simulink model "a1_IEEE9_D"  (R2019a)
settings: Solver=ode23tb  StartTime=-1  StopTime=60  MaxStep=1/60  RelTol=1e-4  AbsTol=1e-3  EnableMultiTasking=on
InitFcn:
  | PSSMODEL=1;
  | MB=[1   0.2 30   1.25 40    12 160];
  | 
  | k=[8.3222    2.6014   19.0811    1.9818    3.6841   19.1783  240.6785    2.5684    4.3666   58.7391 7.6960   47.7975    8.7139  296.2463    2.7543    6.5051   47.7755    0.4780   35.4950   18.1866 94.2186]
  | k1=k(1);
  | k2=k(2);
  | k3=k(3);
  | k4=k(4);
  | k5=k(5);
  | k6=k(6);
  | k7=k(7);
  | k8=k(8);
  | k9=k(9);
  | k10=k(10);
  | k11=k(11);
  | k12=k(12);
  | k13=k(13);
  | k14=k(14);
  | k15=k(15);
  | k16=k(16);
  | k17=k(17);
  | k18=k(18);
  | k19=k(19);
  | k20=k(20);
  | k21=k(21);
values from neighbouring files (symbols this model uses):
  H1 = 2.444444*syn_s    (= 0.479111024)    [a1_IEEE9bus.m]    (also in calc_criticaltime9buses.m = 0.4888888; calc_criticaltime_10inertias.m = 2.444444; calc_nadir_support.m = 2.444444*syn_s; calc_nadirltime_10inertias.m = 2.444444)
  H2 = 5*syn_s    (= 0.98)    [a1_IEEE9bus.m]    (also in calc_criticaltime9buses.m = 1; calc_criticaltime_10inertias.m = 5; calc_nadir_support.m = 5*syn_s; calc_nadirltime_10inertias.m = 5)
  H3 = 5*syn_s    (= 0.98)    [a1_IEEE9bus.m]    (also in calc_criticaltime9buses.m = 1; calc_criticaltime_10inertias.m = 5; calc_nadir_support.m = 5*syn_s; calc_nadirltime_10inertias.m = 5)
  R1 = 0.05    [a1_IEEE9bus.m]    (also in calc_criticaltime9buses.m; calc_criticaltime_10inertias.m; calc_nadir_support.m; calc_nadirltime_10inertias.m)
  R2 = R1    (= 0.05)    [a1_IEEE9bus.m]    (also in calc_criticaltime9buses.m; calc_criticaltime_10inertias.m; calc_nadir_support.m; calc_nadirltime_10inertias.m)
  R3 = R2    (= 0.05)    [a1_IEEE9bus.m]    (also in calc_criticaltime9buses.m; calc_criticaltime_10inertias.m; calc_nadir_support.m; calc_nadirltime_10inertias.m)
  un = 0.30    (= 0.3)    [a1_IEEE9bus.m]    (also in calc_criticaltime9buses.m = 0.4; calc_criticaltime_10inertias.m; calc_nadir_support.m; calc_nadirltime_10inertias.m = 0.2)
undefined symbols (not defined in the file or in its folder): A, B, C, Dd, j
libraries: powerlib x53, sps_avr x3, powerlib_meascontrol x1, simulink x1
(part 1 of 2)
settings Model: Creator=jp536285  LastModifiedBy=Alejandro
settings SolverCC: AutoScaleAbsTol=off
settings DataIOCC: LimitDataPoints=on  SaveFormat=Array  ReturnWorkspaceOutputs=off
settings OptimizationCC: LifeSpan=inf
settings DebuggingCC: UnderspecifiedInitializationDetection=Classic  MergeDetectMultiDrivingBlocksExec=none  SolverPrmCheckMsg=warning  UnconnectedInputMsg=none  UnconnectedOutputMsg=none  UnconnectedLineMsg=none  StateNameClashWarn=warning  SFUnexpectedBacktrackingDiag=warning  SFNoUnconditionalDefaultTransitionDiag=warning  ArithmeticOperatorsInVariantConditions=warning
settings HardwareCC: ProdBitPerPointer=32  ProdBitPerSizeT=32  ProdBitPerPtrDiffT=32  ProdLargestAtomicFloat=None  ProdIntDivRoundTo=Undefined  ProdEndianess=Unspecified  ProdWordSize=32  ProdHWDeviceType=32-bit Generic
settings ModelReferenceCC: PropagateSignalLabelsOutOfModel=off
settings SFSimCC: SimUseLocalCustomCode=off
settings RTWCC: RTWUseLocalCustomCode=off
settings CodeAppCC: StateflowObjectComments=on
settings GRTTargetCC: TargetLangStandard=C89/C90 (ANSI)  GeneratePreprocessorConditionals=Disable all
settings ConfigComp: CovMetricSettings=dw  CovHtmlReporting=on  CovSaveCumulativeToWorkspaceVar=on  CovSaveSingleToWorkspaceVar=on  CovExternalEMLEnable=off
settings SimscapeCC: SimscapeNormalizeSystem=off

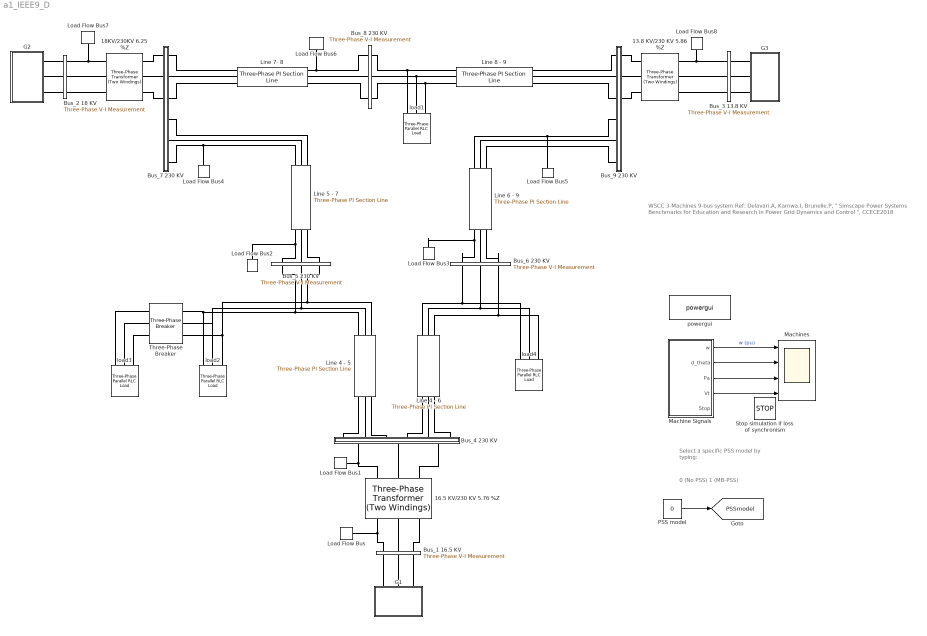
== system a1_IEEE9_D ==
  note: WSCC 3-Machines 9-bus system
      | Ref: Delavari.A, Kamwa.I, Brunelle.P, " Simscape Power Systems Benchmarks for Education
      | and Research in Power Grid Dynamics and Control ", CCECE2018
  note: Select a specific PSS model
      | by typing:
  note: 0  (No PSS)
      | 1  (MB-PSS)
  " Line 4 - 6" : powerlib/Elements/Three-Phase PI Section Line  LConnTagsString=a|b|c  RConnTagsString=A|B|C  Frequency=50  Resistances=[ 9.24e-2 9.24e-1]  Inductances=[ 1.33e-3 3.98e-3]  Capacitances=[8.14e-9 4.88e-9]  Length=97.336  mask(Three-Phase PI Section Line){}
      settings: SourceProductName=Simscape Electrical
      mask Display:
      | % This is a new mask on top of the base mask.
      | % Use "View base mask" link below to see the base mask.
      | patch([0.0 0.0 1 1 0.0 0.0 ],[0.4 0.7 0.7 0.4 0.4 0.7],[0 0 1]);
      | patch([0.4 0.4 0.42 0.42],[0.4 0.75 0.75 0.4],[1 0 0]);
      | patch([0.38 0.38 0.57 0.57],[0.7 0.75 0.75 0.7],[1 0 0]);
      | patch([0.53 0.53 0.55 0.55],[0.4 0.75 0.75 0.4],[1 0 0]);
  " Line 6 - 9" : powerlib/Elements/Three-Phase PI Section Line  LConnTagsString=a|b|c  RConnTagsString=A|B|C  Frequency=50  Resistances=[1.15 1.15e-1]  Inductances=[1.33e-3 3.98e-3]  Capacitances=[9.98e-9 5.99e-9]  Length=179.86  mask(Three-Phase PI Section Line){}
      settings: SourceProductName=Simscape Electrical
      mask Display:
      | % This is a new mask on top of the base mask.
      | % Use "View base mask" link below to see the base mask.
      | patch([0.0 0.0 1 1 0.0 0.0 ],[0.4 0.7 0.7 0.4 0.4 0.7],[0 0 1]);
      | patch([0.4 0.4 0.42 0.42],[0.4 0.75 0.75 0.4],[1 0 0]);
      | patch([0.38 0.38 0.57 0.57],[0.7 0.75 0.75 0.7],[1 0 0]);
      | patch([0.53 0.53 0.55 0.55],[0.4 0.75 0.75 0.4],[1 0 0]);
  13.8 KV/230 KV 5.86 %Z : powerlib/Elements/Three-Phase Transformer (Two Windings)  Winding1Connection=Yg  Winding2Connection=Yg  CoreType=Three single-phase transformers  SetSaturation=off  Hysteresis=off  DataFile='hysteresis'  SetInitialFlux=off  Measurements=None  UNITS=pu  NominalPower=[ 100e6 , 50 ]  Winding1=[ 13.8e3 , 1e-6 , 0 ]  Winding2=[ 230e3 , 1e-6, 0.0586 ]  Rm=500  Lm=500  L0=0.5  Saturation=[ 0,0 ; 0.0024,1.2 ; 1.0,1.52 ]  InitialFluxes=[ 0.8 , -0.8 , 0.7 ]  BreakLoop=off  DiscreteSolver=Trapezoidal iterative  DataType=off  TransfoNumber=1
      settings: SourceProductName=Simscape Electrical
  "16.5 KV/230 KV 5.76 %Z     " : powerlib/Elements/Three-Phase Transformer (Two Windings)  Winding1Connection=Yg  Winding2Connection=Yg  CoreType=Three single-phase transformers  SetSaturation=off  Hysteresis=off  DataFile='hysteresis'  SetInitialFlux=off  Measurements=None  UNITS=pu  NominalPower=[ 100e6 , 50 ]  Winding1=[ 16.5e3 , 1e-6, 0 ]  Winding2=[ 230e3 ,1e-6, 0.0576 ]  Rm=500  Lm=500  L0=0.5  Saturation=[ 0,0 ; 0.0024,1.2 ; 1.0,1.52 ]  InitialFluxes=[ 0.8 , -0.8 , 0.7 ]  BreakLoop=off  DiscreteSolver=Trapezoidal iterative  DataType=off  TransfoNumber=1
      settings: SourceProductName=Simscape Electrical
  18KV/230KV 6.25 %Z : powerlib/Elements/Three-Phase Transformer (Two Windings)  Winding1Connection=Yg  Winding2Connection=Yg  CoreType=Three single-phase transformers  SetSaturation=off  Hysteresis=off  DataFile='hysteresis'  SetInitialFlux=off  Measurements=None  UNITS=pu  NominalPower=[ 100e6 , 50 ]  Winding1=[ 18e3 , 1e-6 , 0]  Winding2=[ 230e3 , 1e-6, 0.0625 ]  Rm=500  Lm=500  L0=0.5  Saturation=[ 0,0 ; 0.0024,1.2 ; 1.0,1.52 ]  InitialFluxes=[ 0.8 , -0.8 , 0.7 ]  BreakLoop=off  DiscreteSolver=Trapezoidal iterative  DataType=off  TransfoNumber=1
      settings: SourceProductName=Simscape Electrical
  Bus_1 16.5 KV : powerlib/Measurements/Three-Phase V-I Measurement  VoltageMeasurement=phase-to-ground  SetLabelV=on  LabelV=Vabc_1  Vpu=on  VpuLL=off  CurrentMeasurement=yes  SetLabelI=on  LabelI=Iabc_1  Ipu=on  Pbase=100e6  Vbase=16.5e3  OutputType=Complex  PhasorSimulation=on  PSBequivalent=0
      settings: SourceProductName=Simscape Electrical
  Bus_2 18 KV : powerlib/Measurements/Three-Phase V-I Measurement  VoltageMeasurement=phase-to-ground  SetLabelV=on  LabelV=Vabc_2  Vpu=on  VpuLL=off  CurrentMeasurement=yes  SetLabelI=on  LabelI=Iabc_2  Ipu=on  Pbase=100e6  Vbase=18e3  OutputType=Complex  PhasorSimulation=on  PSBequivalent=0
      settings: SourceProductName=Simscape Electrical
  Bus_3 13.8 KV : powerlib/Measurements/Three-Phase V-I Measurement  VoltageMeasurement=phase-to-ground  SetLabelV=on  LabelV=Vabc_3  Vpu=on  VpuLL=off  CurrentMeasurement=yes  SetLabelI=on  LabelI=Iabc_3  Ipu=on  Pbase=100e6  Vbase=13.8e3  OutputType=Complex  PhasorSimulation=on  PSBequivalent=0
      settings: SourceProductName=Simscape Electrical
  Bus_4 230 KV : Subsystem
  Bus_5 230 KV : powerlib/Measurements/Three-Phase V-I Measurement  VoltageMeasurement=phase-to-ground  SetLabelV=on  LabelV=Vabc_5  Vpu=on  VpuLL=off  CurrentMeasurement=yes  SetLabelI=on  LabelI=Iabc_5  Ipu=on  Pbase=100e6  Vbase=230e3  OutputType=Complex  PhasorSimulation=on  PSBequivalent=0
      settings: SourceProductName=Simscape Electrical
  Bus_6 230 KV : powerlib/Measurements/Three-Phase V-I Measurement  VoltageMeasurement=phase-to-phase  SetLabelV=on  LabelV=Vabc_6  Vpu=off  VpuLL=on  CurrentMeasurement=yes  SetLabelI=on  LabelI=Iabc_6  Ipu=on  Pbase=100e6  Vbase=230e3  OutputType=Complex  PhasorSimulation=on  PSBequivalent=0
      settings: SourceProductName=Simscape Electrical
  Bus_7 230 KV : Subsystem
  Bus_8 230 KV : powerlib/Measurements/Three-Phase V-I Measurement  VoltageMeasurement=phase-to-phase  SetLabelV=on  LabelV=Vabc_8  Vpu=off  VpuLL=on  CurrentMeasurement=yes  SetLabelI=on  LabelI=Iabc_8  Ipu=on  Pbase=100e6  Vbase=230e3  OutputType=Complex  PhasorSimulation=on  PSBequivalent=0
      settings: SourceProductName=Simscape Electrical
  Bus_9 230 KV : Subsystem
  G1 : Subsystem
  G2 : Subsystem
  G3 : Subsystem
  "Line 4 - 5 " : powerlib/Elements/Three-Phase PI Section Line  LConnTagsString=a|b|c  RConnTagsString=A|B|C  Frequency=50  Resistances=[ 5.88e-2 5.88e-1]  Inductances=[ 1.33e-3 3.98e-3]  Capacitances=[9.81e-9 3.98e-3]  Length=89.93  mask(Three-Phase PI Section Line){}
      settings: SourceProductName=Simscape Electrical
      mask Display:
      | % This is a new mask on top of the base mask.
      | % Use "View base mask" link below to see the base mask.
      | patch([0.0 0.0 1 1 0.0 0.0 ],[0.4 0.7 0.7 0.4 0.4 0.7],[0 0 1]);
      | patch([0.4 0.4 0.42 0.42],[0.4 0.75 0.75 0.4],[1 0 0]);
      | patch([0.38 0.38 0.57 0.57],[0.7 0.75 0.75 0.7],[1 0 0]);
      | patch([0.53 0.53 0.55 0.55],[0.4 0.75 0.75 0.4],[1 0 0]);
  "Line 5 - 7 " : powerlib/Elements/Three-Phase PI Section Line  LConnTagsString=a|b|c  RConnTagsString=A|B|C  Frequency=50  Resistances=[9.94e-2 9.94e-1]  Inductances=[1.33e-3 3.98e-3]  Capacitances=[9.01e-9 5.41e-9]  Length=170.338  mask(Three-Phase PI Section Line){}
      settings: SourceProductName=Simscape Electrical
      mask Display:
      | % This is a new mask on top of the base mask.
      | % Use "View base mask" link below to see the base mask.
      | patch([0.0 0.0 1 1 0.0 0.0 ],[0.4 0.7 0.7 0.4 0.4 0.7],[0 0 1]);
      | patch([0.4 0.4 0.42 0.42],[0.4 0.75 0.75 0.4],[1 0 0]);
      | patch([0.38 0.38 0.57 0.57],[0.7 0.75 0.75 0.7],[1 0 0]);
      | patch([0.53 0.53 0.55 0.55],[0.4 0.75 0.75 0.4],[1 0 0]);
  Line 7- 8 : powerlib/Elements/Three-Phase PI Section Line  LConnTagsString=a|b|c  RConnTagsString=A|B|C  Frequency=50  Resistances=[5.9e-2 5.9e-1]  Inductances=[1.33e-3 3.98e-3]  Capacitances=[9.81e-9 5.89e-9]  Length=76.176  mask(Three-Phase PI Section Line){}
      settings: SourceProductName=Simscape Electrical
      mask Display:
      | % This is a new mask on top of the base mask.
      | % Use "View base mask" link below to see the base mask.
      | patch([0.0 0.0 1 1 0.0 0.0 ],[0.4 0.7 0.7 0.4 0.4 0.7],[0 0 1]);
      | patch([0.4 0.4 0.42 0.42],[0.4 0.75 0.75 0.4],[1 0 0]);
      | patch([0.38 0.38 0.57 0.57],[0.7 0.75 0.75 0.7],[1 0 0]);
      | patch([0.53 0.53 0.55 0.55],[0.4 0.75 0.75 0.4],[1 0 0]);
  Line 8 - 9 : powerlib/Elements/Three-Phase PI Section Line  LConnTagsString=a|b|c  RConnTagsString=A|B|C  Frequency=50  Resistances=[5.9e-2 5.9e-1]  Inductances=[1.33e-3 3.98e-3]  Capacitances=[9.83e-9 5.9e-9]  Length=106.649  mask(Three-Phase PI Section Line){}
      settings: SourceProductName=Simscape Electrical
      mask Display:
      | % This is a new mask on top of the base mask.
      | % Use "View base mask" link below to see the base mask.
      | patch([0.0 0.0 1 1 0.0 0.0 ],[0.4 0.7 0.7 0.4 0.4 0.7],[0 0 1]);
      | patch([0.4 0.4 0.42 0.42],[0.4 0.75 0.75 0.4],[1 0 0]);
      | patch([0.38 0.38 0.57 0.57],[0.7 0.75 0.75 0.7],[1 0 0]);
      | patch([0.53 0.53 0.55 0.55],[0.4 0.75 0.75 0.4],[1 0 0]);
  Load Flow Bus : powerlib/Measurements/Load Flow Bus  LConnTagsString=a  Phases=single  Connectors=on one side  ID=BUS_1  Vbase=16.5e3  Vref=1.04  Vangle=0  VLF=1.04  VLFb=1  VLFc=1  angleLF=0  angleLFb=0  angleLFc=0
      settings: AttributesFormatString=%<ID>\n%<Vbase>V\n%<VLF>pu\n%<angleLF>deg.  SourceProductName=Simscape Electrical
  Load Flow Bus1 : powerlib/Measurements/Load Flow Bus  LConnTagsString=a  Phases=single  Connectors=on one side  ID=BUS_4  Vbase=230e3  Vref=1  Vangle=0  VLF=1.021  VLFb=1  VLFc=1  angleLF=-2.239  angleLFb=0  angleLFc=0
      settings: AttributesFormatString=%<ID>\n%<Vbase>V\n%<VLF>pu\n%<angleLF>deg.  SourceProductName=Simscape Electrical
  Load Flow Bus2 : powerlib/Measurements/Load Flow Bus  LConnTagsString=a  Phases=single  Connectors=on one side  ID=BUS_5  Vbase=230e3  Vref=1  Vangle=0  VLF=0.9938  VLFb=1  VLFc=1  angleLF=-3.685  angleLFb=0  angleLFc=0
      settings: AttributesFormatString=%<ID>\n%<Vbase>V\n%<VLF>pu\n%<angleLF>deg.  SourceProductName=Simscape Electrical
  Load Flow Bus3 : powerlib/Measurements/Load Flow Bus  LConnTagsString=a  Phases=single  Connectors=on one side  ID=BUS_6  Vbase=230e3  Vref=1  Vangle=0  VLF=1.007  VLFb=1  VLFc=1  angleLF=-3.444  angleLFb=0  angleLFc=0
      settings: AttributesFormatString=%<ID>\n%<Vbase>V\n%<VLF>pu\n%<angleLF>deg.  SourceProductName=Simscape Electrical
  Load Flow Bus4 : powerlib/Measurements/Load Flow Bus  LConnTagsString=a  Phases=single  Connectors=on one side  ID=BUS_7  Vbase=230e3  Vref=1  Vangle=0  VLF=1.024  VLFb=1  VLFc=1  angleLF=2.693  angleLFb=0  angleLFc=0
      settings: AttributesFormatString=%<ID>\n%<Vbase>V\n%<VLF>pu\n%<angleLF>deg.  SourceProductName=Simscape Electrical
  Load Flow Bus5 : powerlib/Measurements/Load Flow Bus  LConnTagsString=a  Phases=single  Connectors=on one side  ID=BUS_9  Vbase=230e3  Vref=1  Vangle=0  VLF=1.029  VLFb=1  VLFc=1  angleLF=1.226  angleLFb=0  angleLFc=0
      settings: AttributesFormatString=%<ID>\n%<Vbase>V\n%<VLF>pu\n%<angleLF>deg.  SourceProductName=Simscape Electrical
  Load Flow Bus6 : powerlib/Measurements/Load Flow Bus  LConnTagsString=a  Phases=single  Connectors=on one side  ID=BUS_8  Vbase=230e3  Vref=1  Vangle=0  VLF=1.014  VLFb=1  VLFc=1  angleLF=0.2062  angleLFb=0  angleLFc=0
      settings: AttributesFormatString=%<ID>\n%<Vbase>V\n%<VLF>pu\n%<angleLF>deg.  SourceProductName=Simscape Electrical
  Load Flow Bus7 : powerlib/Measurements/Load Flow Bus  LConnTagsString=a  Phases=single  Connectors=on one side  ID=BUS_2  Vbase=18e3  Vref=1.025  Vangle=0  VLF=1.025  VLFb=1  VLFc=1  angleLF=8.256  angleLFb=0  angleLFc=0
      settings: AttributesFormatString=%<ID>\n%<Vbase>V\n%<VLF>pu\n%<angleLF>deg.  SourceProductName=Simscape Electrical
  Load Flow Bus8 : powerlib/Measurements/Load Flow Bus  LConnTagsString=a  Phases=single  Connectors=on one side  ID=BUS_3  Vbase=13.8e3  Vref=1.025  Vangle=0  VLF=1.025  VLFb=1  VLFc=1  angleLF=3.927  angleLFb=0  angleLFc=0
      settings: AttributesFormatString=%<ID>\n%<Vbase>V\n%<VLF>pu\n%<angleLF>deg.  SourceProductName=Simscape Electrical
  Machine Signals : Subsystem
  Machines : Scope  NumInputPorts=4
  PSS model : Constant  Value=0
  Stop simulation if loss of synchronism : Stop
  Three-Phase Breaker : powerlib/Elements/Three-Phase Breaker  InitialState=open  SwitchA=on  SwitchB=on  SwitchC=on  SwitchTimes=0  External=off  BreakerResistance=0.00001  SnubberResistance=1e9  SnubberCapacitance=inf  Measurements=None
      settings: SourceProductName=Simscape Electrical
  load1 : powerlib/Elements/Three-Phase Parallel RLC Load  LConnTagsString=A|B|C  Configuration=Y (grounded)  NominalVoltage=(230000)*1.01415  Vabc=[1e3 1e3 1e3]  Vabcp=[1e3 1e3 1e3]  NominalFrequency=50  UnbalancedPower=off  ActivePower=100e6  InductivePower=35e6  CapacitivePower=0  Pabc=[10e3 9e3 11e3]  QLabc=[100 90 110]  QCabc=[100 90 110]  Pabcp=[10e3 9e3 11e3]  QLabcp=[100 90 110]  QCabcp=[100 90 110]  Measurements=None  LoadType=constant PQ
      settings: SourceProductName=Simscape Electrical
  load2 : powerlib/Elements/Three-Phase Parallel RLC Load  LConnTagsString=A|B|C  Configuration=Y (grounded)  NominalVoltage=(230000)*0.993797  Vabc=[1e3 1e3 1e3]  Vabcp=[1e3 1e3 1e3]  NominalFrequency=50  UnbalancedPower=off  ActivePower=125e6  InductivePower=50e6  CapacitivePower=0  Pabc=[10e3 9e3 11e3]  QLabc=[100 90 110]  QCabc=[100 90 110]  Pabcp=[10e3 9e3 11e3]  QLabcp=[100 90 110]  QCabcp=[100 90 110]  Measurements=None  LoadType=constant PQ
      settings: SourceProductName=Simscape Electrical
  load3 : powerlib/Elements/Three-Phase Parallel RLC Load  LConnTagsString=A|B|C  Configuration=Y (grounded)  NominalVoltage=(230000)*0.993797  Vabc=[1e3 1e3 1e3]  Vabcp=[1e3 1e3 1e3]  NominalFrequency=50  UnbalancedPower=off  ActivePower=(315e6)*un  InductivePower=0  CapacitivePower=0  Pabc=[10e3 9e3 11e3]  QLabc=[100 90 110]  QCabc=[100 90 110]  Pabcp=[10e3 9e3 11e3]  QLabcp=[100 90 110]  QCabcp=[100 90 110]  Measurements=None  LoadType=constant PQ
      settings: SourceProductName=Simscape Electrical
  load4 : powerlib/Elements/Three-Phase Parallel RLC Load  LConnTagsString=A|B|C  Configuration=Y (grounded)  NominalVoltage=(230000)*1.00721  Vabc=[1e3 1e3 1e3]  Vabcp=[1e3 1e3 1e3]  NominalFrequency=50  UnbalancedPower=off  ActivePower=9e+07  InductivePower=3e+07  CapacitivePower=0  Pabc=[10e3 9e3 11e3]  QLabc=[100 90 110]  QCabc=[100 90 110]  Pabcp=[10e3 9e3 11e3]  QLabcp=[100 90 110]  QCabcp=[100 90 110]  Measurements=None  LoadType=constant PQ
      settings: SourceProductName=Simscape Electrical
  powergui : powerlib/powergui  Priority=1  SimulationMode=Phasor  SampleTime=50e-6  frequency=50  Iterations=50  frequencyindice=50  Pbase=10e7  ErrMax=1e-05  UnitsV=kV  UnitsW=MW  buscounter=0  FunctionMessages=off  echomessages=off  EnableUseOfTLC=off  CurrentSourceSwitches=off  DisableSnubberDevices=off  DisableRonSwitches=off  DisableVfSwitches=off  DisplayEquations=off  AutomaticDiscreteSolvers=off  SolverType=Tustin  Interpol=off  ExternalGateDelay=off  methode=off  Ts=0  x0status=steady  SPID=off  SwTol=0  HookPort=off  NonlinearTolerance=0  nMaxIteration=15  ContinueOnMaxIteration=off  RestoreLinks=warning  ResistiveCurrentMeasurement=off  Frange=[0:2:500]  Ylog=off  Xlog=on  ShowGrid=off  save=off  variable=ZData  structure=0  ZoomFFT=off  StartTime=0.0  cycles=1  DisplayStyle=1  fundamental=60  FreqAxis=off  MaxFrequency=1000  frequencyindicesteady=1  RmsSteady=1  display=off
      settings: SourceProductName=Simscape Electrical
  tag scope: PSSmodel=global
  wires:
  Machine Signals/1(w) -> Machines/1  "w (pu)"
  Machine Signals/2(d_theta) -> Machines/2
  Machine Signals/3(Pa) -> Machines/3
  Machine Signals/4(Vt) -> Machines/4
  PSS model/1 -> [PSSmodel]
  connections:
  G2/LConn2 -- Bus_2 18 KV/LConn2
  18KV/230KV 6.25 %Z/LConn2 -- Bus_2 18 KV/RConn2
  18KV/230KV 6.25 %Z/RConn2 -- Bus_7 230 KV/LConn2
  Bus_2 18 KV/RConn1 -- 18KV/230KV 6.25 %Z/LConn1 -- Load Flow Bus7/LConn1
  Bus_2 18 KV/RConn3 -- 18KV/230KV 6.25 %Z/LConn3
  Bus_7 230 KV/LConn1 -- 18KV/230KV 6.25 %Z/RConn1
  18KV/230KV 6.25 %Z/RConn3 -- Bus_7 230 KV/LConn3
  Load Flow Bus8/LConn1 -- 13.8 KV/230 KV 5.86 %Z/LConn1 -- Bus_3 13.8 KV/LConn1
  13.8 KV/230 KV 5.86 %Z/LConn2 -- Bus_3 13.8 KV/LConn2
  13.8 KV/230 KV 5.86 %Z/LConn3 -- Bus_3 13.8 KV/LConn3
  Bus_1 16.5 KV/LConn1 -- Load Flow Bus/LConn1 -- "16.5 KV/230 KV 5.76 %Z     "/LConn1
  Bus_1 16.5 KV/LConn3 -- "16.5 KV/230 KV 5.76 %Z     "/LConn3
  Bus_1 16.5 KV/LConn2 -- "16.5 KV/230 KV 5.76 %Z     "/LConn2
  13.8 KV/230 KV 5.86 %Z/RConn1 -- Bus_9 230 KV/RConn1
  13.8 KV/230 KV 5.86 %Z/RConn2 -- Bus_9 230 KV/RConn2
  13.8 KV/230 KV 5.86 %Z/RConn3 -- Bus_9 230 KV/RConn3
  Bus_4 230 KV/LConn1 -- "16.5 KV/230 KV 5.76 %Z     "/RConn1 -- Load Flow Bus1/LConn1
  Bus_4 230 KV/LConn2 -- "16.5 KV/230 KV 5.76 %Z     "/RConn2
  Line 8 - 9/LConn1 -- load1/LConn1 -- Bus_8 230 KV/LConn1
  Bus_8 230 KV/LConn2 -- load1/LConn2 -- Line 8 - 9/LConn2
  Line 8 - 9/LConn3 -- load1/LConn3 -- Bus_8 230 KV/LConn3
  "16.5 KV/230 KV 5.76 %Z     "/RConn3 -- Bus_4 230 KV/LConn3
  "Line 4 - 5 "/LConn1 -- Bus_5 230 KV/RConn1 -- load2/LConn1 -- Three-Phase Breaker/RConn1
  "Line 4 - 5 "/LConn2 -- Three-Phase Breaker/RConn2 -- load2/LConn2 -- Bus_5 230 KV/RConn2
  "Line 4 - 5 "/LConn3 -- Bus_5 230 KV/RConn3 -- Three-Phase Breaker/RConn3 -- load2/LConn3
  " Line 4 - 6"/LConn1 -- load4/LConn1 -- Bus_6 230 KV/RConn1
  " Line 4 - 6"/LConn2 -- load4/LConn2 -- Bus_6 230 KV/RConn2
  " Line 4 - 6"/LConn3 -- load4/LConn3 -- Bus_6 230 KV/RConn3
  Line 7- 8/LConn1 -- Bus_7 230 KV/RConn1
  Line 7- 8/LConn2 -- Bus_7 230 KV/RConn2
  Bus_7 230 KV/RConn3 -- Line 7- 8/LConn3
  Bus_8 230 KV/RConn1 -- Load Flow Bus6/LConn1 -- Line 7- 8/RConn1
  Line 7- 8/RConn2 -- Bus_8 230 KV/RConn2
  Line 7- 8/RConn3 -- Bus_8 230 KV/RConn3
  Line 8 - 9/RConn2 -- Bus_9 230 KV/LConn2
  Line 8 - 9/RConn1 -- Bus_9 230 KV/LConn1
  Line 8 - 9/RConn3 -- Bus_9 230 KV/LConn3
  "Line 5 - 7 "/RConn1 -- Bus_5 230 KV/LConn1 -- Load Flow Bus2/LConn1
  "Line 5 - 7 "/RConn2 -- Bus_5 230 KV/LConn2
  "Line 5 - 7 "/RConn3 -- Bus_5 230 KV/LConn3
  "Line 5 - 7 "/LConn1 -- Load Flow Bus4/LConn1 -- Bus_7 230 KV/RConn6
  "Line 5 - 7 "/LConn2 -- Bus_7 230 KV/RConn5
  "Line 5 - 7 "/LConn3 -- Bus_7 230 KV/RConn4
  " Line 6 - 9"/RConn1 -- Load Flow Bus5/LConn1 -- Bus_9 230 KV/LConn4
  Bus_9 230 KV/LConn5 -- " Line 6 - 9"/RConn2
  Bus_6 230 KV/LConn1 -- Load Flow Bus3/LConn1 -- " Line 6 - 9"/LConn1
  Bus_6 230 KV/LConn2 -- " Line 6 - 9"/LConn2
  Bus_6 230 KV/LConn3 -- " Line 6 - 9"/LConn3
  " Line 6 - 9"/RConn3 -- Bus_9 230 KV/LConn6
  "Line 4 - 5 "/RConn2 -- Bus_4 230 KV/RConn2
  "Line 4 - 5 "/RConn1 -- Bus_4 230 KV/RConn1
  "Line 4 - 5 "/RConn3 -- Bus_4 230 KV/RConn3
  " Line 4 - 6"/RConn2 -- Bus_4 230 KV/RConn5
  " Line 4 - 6"/RConn1 -- Bus_4 230 KV/RConn4
  " Line 4 - 6"/RConn3 -- Bus_4 230 KV/RConn6
  G3/LConn1 -- Bus_3 13.8 KV/RConn1
  G3/LConn2 -- Bus_3 13.8 KV/RConn2
  G3/LConn3 -- Bus_3 13.8 KV/RConn3
  G2/LConn3 -- Bus_2 18 KV/LConn3
  G2/LConn1 -- Bus_2 18 KV/LConn1
  G1/LConn1 -- Bus_1 16.5 KV/RConn1
  G1/LConn2 -- Bus_1 16.5 KV/RConn2
  G1/LConn3 -- Bus_1 16.5 KV/RConn3
  load3/LConn1 -- Three-Phase Breaker/LConn1
  load3/LConn2 -- Three-Phase Breaker/LConn2
  load3/LConn3 -- Three-Phase Breaker/LConn3

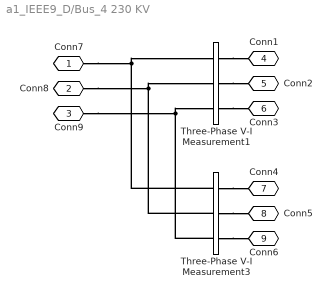
== system a1_IEEE9_D/Bus_4 230 KV ==
  Three-Phase V-I Measurement1 : powerlib/Measurements/Three-Phase V-I Measurement  VoltageMeasurement=phase-to-ground  SetLabelV=on  LabelV=Vabc_45  Vpu=on  VpuLL=off  CurrentMeasurement=yes  SetLabelI=on  LabelI=Iabc_45  Ipu=on  Pbase=100e6  Vbase=230e3  OutputType=Complex  PhasorSimulation=on  PSBequivalent=0
      settings: SourceProductName=Simscape Electrical
  Three-Phase V-I Measurement3 : powerlib/Measurements/Three-Phase V-I Measurement  VoltageMeasurement=phase-to-ground  SetLabelV=on  LabelV=Vabc_46  Vpu=on  VpuLL=off  CurrentMeasurement=yes  SetLabelI=on  LabelI=Iabc_46  Ipu=on  Pbase=100e6  Vbase=230e3  OutputType=Complex  PhasorSimulation=on  PSBequivalent=0
      settings: SourceProductName=Simscape Electrical
  Conn7 : PMIOPort  Side=Left
  Conn8 : PMIOPort  Port=2  Side=Left
  Conn9 : PMIOPort  Port=3  Side=Left
  Conn1 : PMIOPort  Port=4  Side=Right
  Conn2 : PMIOPort  Port=5  Side=Right
  Conn3 : PMIOPort  Port=6  Side=Right
  Conn4 : PMIOPort  Port=7  Side=Right
  Conn5 : PMIOPort  Port=8  Side=Right
  Conn6 : PMIOPort  Port=9  Side=Right
  connections:
  Three-Phase V-I Measurement3/LConn3 -- Conn9/RConn1 -- Three-Phase V-I Measurement1/LConn3
  Three-Phase V-I Measurement3/LConn2 -- Conn8/RConn1 -- Three-Phase V-I Measurement1/LConn2
  Three-Phase V-I Measurement3/LConn1 -- Conn7/RConn1 -- Three-Phase V-I Measurement1/LConn1
  Three-Phase V-I Measurement3/RConn3 -- Conn6/RConn1
  Three-Phase V-I Measurement1/RConn3 -- Conn3/RConn1
  Three-Phase V-I Measurement1/RConn1 -- Conn1/RConn1
  Three-Phase V-I Measurement1/RConn2 -- Conn2/RConn1
  Three-Phase V-I Measurement3/RConn1 -- Conn4/RConn1
  Three-Phase V-I Measurement3/RConn2 -- Conn5/RConn1

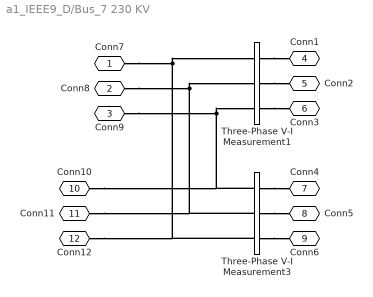
== system a1_IEEE9_D/Bus_7 230 KV ==
  Three-Phase V-I Measurement1 : powerlib/Measurements/Three-Phase V-I Measurement  VoltageMeasurement=phase-to-ground  SetLabelV=on  LabelV=Vabc_7  Vpu=on  VpuLL=off  CurrentMeasurement=yes  SetLabelI=on  LabelI=Iabc_7  Ipu=on  Pbase=100e6  Vbase=230e3  OutputType=Complex  PhasorSimulation=on  PSBequivalent=0
      settings: SourceProductName=Simscape Electrical
  Three-Phase V-I Measurement3 : powerlib/Measurements/Three-Phase V-I Measurement  VoltageMeasurement=phase-to-ground  SetLabelV=on  LabelV=Vab  Vpu=on  VpuLL=off  CurrentMeasurement=yes  SetLabelI=on  LabelI=Iab  Ipu=on  Pbase=100e6  Vbase=230e3  OutputType=Complex  PhasorSimulation=on  PSBequivalent=0
      settings: SourceProductName=Simscape Electrical
  Conn7 : PMIOPort  Side=Left
  Conn8 : PMIOPort  Port=2  Side=Left
  Conn9 : PMIOPort  Port=3  Side=Left
  Conn1 : PMIOPort  Port=4  Side=Right
  Conn2 : PMIOPort  Port=5  Side=Right
  Conn3 : PMIOPort  Port=6  Side=Right
  Conn4 : PMIOPort  Port=7  Side=Right
  Conn5 : PMIOPort  Port=8  Side=Right
  Conn6 : PMIOPort  Port=9  Side=Right
  Conn10 : PMIOPort  Port=10  Side=Left
  Conn11 : PMIOPort  Port=11  Side=Left
  Conn12 : PMIOPort  Port=12  Side=Left
  connections:
  Three-Phase V-I Measurement3/RConn2 -- Conn5/RConn1
  Three-Phase V-I Measurement3/RConn1 -- Conn4/RConn1
  Three-Phase V-I Measurement1/RConn2 -- Conn2/RConn1
  Three-Phase V-I Measurement1/RConn1 -- Conn1/RConn1
  Three-Phase V-I Measurement1/RConn3 -- Conn3/RConn1
  Three-Phase V-I Measurement3/RConn3 -- Conn6/RConn1
  Conn7/RConn1 -- Three-Phase V-I Measurement3/LConn3 -- Conn12/RConn1 -- Three-Phase V-I Measurement1/LConn1
  Conn8/RConn1 -- Three-Phase V-I Measurement3/LConn2 -- Conn11/RConn1 -- Three-Phase V-I Measurement1/LConn2
  Conn9/RConn1 -- Conn10/RConn1 -- Three-Phase V-I Measurement3/LConn1 -- Three-Phase V-I Measurement1/LConn3

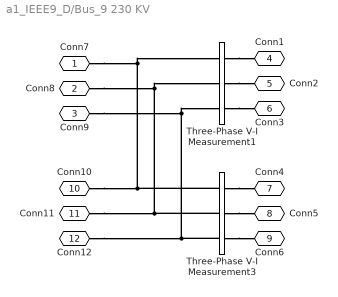
== system a1_IEEE9_D/Bus_9 230 KV ==
  Three-Phase V-I Measurement1 : powerlib/Measurements/Three-Phase V-I Measurement  VoltageMeasurement=phase-to-ground  SetLabelV=on  LabelV=Vabc_9  Vpu=on  VpuLL=off  CurrentMeasurement=yes  SetLabelI=on  LabelI=Iabc_9  Ipu=on  Pbase=100e6  Vbase=230e3  OutputType=Complex  PhasorSimulation=on  PSBequivalent=0
      settings: SourceProductName=Simscape Electrical
  Three-Phase V-I Measurement3 : powerlib/Measurements/Three-Phase V-I Measurement  VoltageMeasurement=phase-to-ground  SetLabelV=on  LabelV=Vabc  Vpu=on  VpuLL=off  CurrentMeasurement=yes  SetLabelI=on  LabelI=Iabc  Ipu=on  Pbase=100e6  Vbase=230e3  OutputType=Complex  PhasorSimulation=on  PSBequivalent=0
      settings: SourceProductName=Simscape Electrical
  Conn7 : PMIOPort  Side=Left
  Conn8 : PMIOPort  Port=2  Side=Left
  Conn9 : PMIOPort  Port=3  Side=Left
  Conn1 : PMIOPort  Port=4  Side=Right
  Conn2 : PMIOPort  Port=5  Side=Right
  Conn3 : PMIOPort  Port=6  Side=Right
  Conn4 : PMIOPort  Port=7  Side=Right
  Conn5 : PMIOPort  Port=8  Side=Right
  Conn6 : PMIOPort  Port=9  Side=Right
  Conn10 : PMIOPort  Port=10  Side=Left
  Conn11 : PMIOPort  Port=11  Side=Left
  Conn12 : PMIOPort  Port=12  Side=Left
  connections:
  Conn12/RConn1 -- Three-Phase V-I Measurement3/LConn3 -- Conn9/RConn1 -- Three-Phase V-I Measurement1/LConn3
  Conn11/RConn1 -- Three-Phase V-I Measurement3/LConn2 -- Conn8/RConn1 -- Three-Phase V-I Measurement1/LConn2
  Conn10/RConn1 -- Three-Phase V-I Measurement3/LConn1 -- Conn7/RConn1 -- Three-Phase V-I Measurement1/LConn1
  Three-Phase V-I Measurement3/RConn3 -- Conn6/RConn1
  Three-Phase V-I Measurement1/RConn3 -- Conn3/RConn1
  Three-Phase V-I Measurement1/RConn1 -- Conn1/RConn1
  Three-Phase V-I Measurement1/RConn2 -- Conn2/RConn1
  Three-Phase V-I Measurement3/RConn1 -- Conn4/RConn1
  Three-Phase V-I Measurement3/RConn2 -- Conn5/RConn1

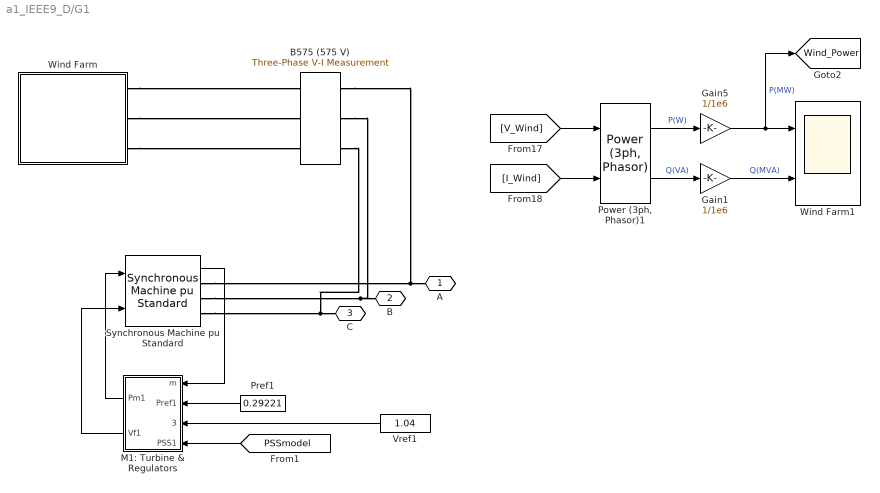
== system a1_IEEE9_D/G1 ==
  B575 (575 V) : powerlib/Measurements/Three-Phase V-I Measurement  VoltageMeasurement=phase-to-ground  SetLabelV=on  LabelV=V_Wind  Vpu=off  VpuLL=off  CurrentMeasurement=yes  SetLabelI=on  LabelI=I_Wind  Ipu=off  Pbase=6*1.5e6/0.9  Vbase=575  OutputType=Complex  PhasorSimulation=on  PSBequivalent=0
      settings: SourceProductName=Simscape Electrical
  Gain1 : Gain  Gain=1/1e6
  Gain5 : Gain  Gain=1/1e6
  M1: Turbine & Regulators : Subsystem
  "Power (3ph, Phasor)1" : powerlib_meascontrol/Measurements/Power (3ph, Phasor)
      settings: SourceProductName=Simscape Electrical  SourceProductBaseCode=PS
  Pref1 : Constant  Value=0.29221
  Synchronous Machine pu Standard : powerlib/Machines/Synchronous Machine pu Standard  PresetModel=No  MechanicalLoad=Mechanical power Pm  ShowDetailedParameters=on  RotorType=Round  Units=per unit standard parameters  MeasurementBus=off  NominalParameters="[247.5e6  16500   50 ]"  Reactances1=[ 1.81, 0.3, 0.23, 1.76, 0.65, 0.25, 0.15 ]  Reactances2=[1.146 .0608 .25 0.0969*10 0.0969 .25 .025]  dAxisTimeConstants=Open-circuit  qAxisTimeConstants=Open-circuit  TimeConstants1=[8.96 0.3 0.31 0.05]  TimeConstants2=[ 8.0, 0.03, 1.0, 0.07 ]  TimeConstants3="[  4.49  0.0681  0.0513  ]"  TimeConstants4=[ 8.0, 0.03, 0.3371, 0.0295 ]  TimeConstants5=[ 1.01, 0.053, 0.1 ]  TimeConstants6=[ 1.3201, 0.023, 1.0, 0.07 ]  TimeConstants7=[0.012 0.003 0.003]  TimeConstants8=[ 1.3201, 0.0231, 0.3371, 0.0295 ]  StatorResistance=0.0025  Mechanical="[ H1  0  4]"  PolePairs=20  InitialConditions=[0 -68.9621 0.312855 0.312855 0.312855 -26.1902 -146.19 93.8098 1.38688]  SetSaturation=off  Saturation=[0.6404,0.7127,0.8441,0.9214,0.9956,1.082,1.19,1.316,1.457;0.7,0.7698,0.8872,0.9466,0.9969,1.046,1.1,1.151,1.201]  LoadFlowParameters=[2 72000000 0 0 0]  TsPowergui=0  TsBlock=-1  IterativeModel=Trapezoidal non iterative  IterativeDiscreteModel=Trapezoidal non iterative  BusType=swing  Pref=0  Qref=0  Qmin=-inf  Qmax=inf  PLF=0  QLF=0
      settings: SourceProductName=Simscape Electrical
  Vref1 : Constant  Value=1.04
  Wind Farm : Subsystem
  Wind Farm1 : Scope  NumInputPorts=2
  A : PMIOPort  Side=Left
  B : PMIOPort  Port=2  Side=Left
  C : PMIOPort  Port=3  Side=Left
  tag scope: Wind_Power=global
  wires:
  Pref1/1 -> M1: Turbine & Regulators/2(Pref1)
  [PSSmodel] -> M1: Turbine & Regulators/4(PSS1)
  M1: Turbine & Regulators/1(Pm1) -> Synchronous Machine pu Standard/1
  M1: Turbine & Regulators/2(Vf1) -> Synchronous Machine pu Standard/2
  Vref1/1 -> M1: Turbine & Regulators/3(Vref1)
  Synchronous Machine pu Standard/1 -> M1: Turbine & Regulators/1(m)
  [V_Wind] -> "Power (3ph, Phasor)1"/1
  "Power (3ph, Phasor)1"/2 -> Gain1/1  "Q(VA)"
  Gain1/1 -> Wind Farm1/2  "Q(MVA)"
  "Power (3ph, Phasor)1"/1 -> Gain5/1  "P(W)"
  [I_Wind] -> "Power (3ph, Phasor)1"/2
  Gain5/1 -> [Wind_Power], Wind Farm1/1  "P(MW)"
  connections:
  Synchronous Machine pu Standard/RConn1 -- B575 (575 V)/RConn1 -- A/RConn1
  Synchronous Machine pu Standard/RConn2 -- B575 (575 V)/RConn2 -- B/RConn1
  Synchronous Machine pu Standard/RConn3 -- B575 (575 V)/RConn3 -- C/RConn1
  Wind Farm/RConn1 -- B575 (575 V)/LConn1
  Wind Farm/RConn2 -- B575 (575 V)/LConn2
  Wind Farm/RConn3 -- B575 (575 V)/LConn3

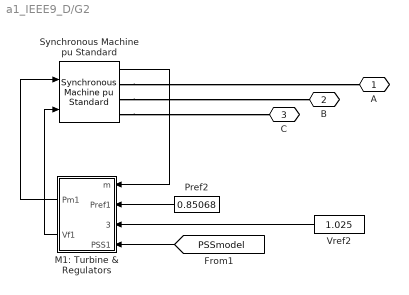
== system a1_IEEE9_D/G2 ==
  M1: Turbine & Regulators : Subsystem
  Pref2 : Constant  Value=0.85068
  Synchronous Machine pu Standard : powerlib/Machines/Synchronous Machine pu Standard  PresetModel=No  MechanicalLoad=Mechanical power Pm  ShowDetailedParameters=on  RotorType=Round  Units=per unit standard parameters  MeasurementBus=off  NominalParameters="[192e6  18000   50 ]"  Reactances1=[0.8958 .1198 .25 1.7 .8645 .1969 .220]  Reactances2=[2.24 0.17 0.12 1.02 0.13 0.08]  dAxisTimeConstants=Open-circuit  qAxisTimeConstants=Open-circuit  TimeConstants1="[ 4.4849  0.0681  0.1  ]"  TimeConstants2=[6 .03 .535 .05]  TimeConstants3="[  4.49  0.0681  0.0513  ]"  TimeConstants4=[ 8.0, 0.03, 0.3371, 0.0295 ]  TimeConstants5=[ 1.01, 0.053, 0.1 ]  TimeConstants6=[ 1.3201, 0.023, 1.0, 0.07 ]  TimeConstants7=[0.012 0.003 0.003]  TimeConstants8=[ 1.3201, 0.0231, 0.3371, 0.0295 ]  StatorResistance=0.0025  Mechanical="[ H2  0  4]"  PolePairs=20  InitialConditions=[0 -30.0411 0.82975 0.82975 0.82975 4.813 -115.187 124.813 1.24637]  SetSaturation=off  Saturation=[0.6404,0.7127,0.8441,0.9214,0.9956,1.082,1.19,1.316,1.457;0.7,0.7698,0.8872,0.9466,0.9969,1.046,1.1,1.151,1.201]  LoadFlowParameters=[1,0,0,0,0]  TsPowergui=0  TsBlock=-1  IterativeModel=Trapezoidal non iterative  IterativeDiscreteModel=Trapezoidal non iterative  BusType=PV  Pref=163e6  Qref=0  Qmin=-inf  Qmax=inf  PLF=0  QLF=0
      settings: SourceProductName=Simscape Electrical
  Vref2 : Constant  Value=1.025
  A : PMIOPort  Side=Left
  B : PMIOPort  Port=2  Side=Left
  C : PMIOPort  Port=3  Side=Left
  wires:
  Pref2/1 -> M1: Turbine & Regulators/2(Pref1)
  [PSSmodel] -> M1: Turbine & Regulators/4(PSS1)
  M1: Turbine & Regulators/1(Pm1) -> Synchronous Machine pu Standard/1
  M1: Turbine & Regulators/2(Vf1) -> Synchronous Machine pu Standard/2
  Synchronous Machine pu Standard/1 -> M1: Turbine & Regulators/1(m)
  Vref2/1 -> M1: Turbine & Regulators/3(Vref1)
  connections:
  Synchronous Machine pu Standard/RConn1 -- A/RConn1
  Synchronous Machine pu Standard/RConn2 -- B/RConn1
  Synchronous Machine pu Standard/RConn3 -- C/RConn1

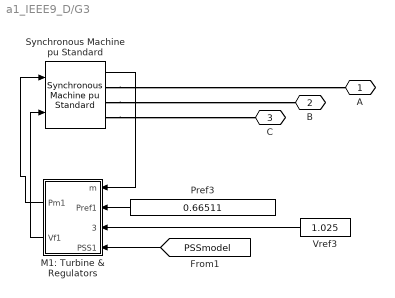
== system a1_IEEE9_D/G3 ==
  M1: Turbine & Regulators : Subsystem
  Pref3 : Constant  Value=0.66511
  Synchronous Machine pu Standard : powerlib/Machines/Synchronous Machine pu Standard  PresetModel=No  MechanicalLoad=Mechanical power Pm  ShowDetailedParameters=on  RotorType=Round  Units=per unit standard parameters  MeasurementBus=off  NominalParameters="[128e6  13800   50 ]"  Reactances1=[1.3125 .1813 .25 1.2578 .25 .25 .246]  Reactances2=[2.24 0.17 0.12 1.02 0.13 0.08]  dAxisTimeConstants=Open-circuit  qAxisTimeConstants=Open-circuit  TimeConstants1="[ 4.4849  0.0681  0.1  ]"  TimeConstants2=[5.89 .03 .6 .05]  TimeConstants3="[  4.49  0.0681  0.0513  ]"  TimeConstants4=[ 8.0, 0.03, 0.3371, 0.0295 ]  TimeConstants5=[ 1.01, 0.053, 0.1 ]  TimeConstants6=[ 1.3201, 0.023, 1.0, 0.07 ]  TimeConstants7=[0.012 0.003 0.003]  TimeConstants8=[ 1.3201, 0.0231, 0.3371, 0.0295 ]  StatorResistance=0.0025  Mechanical="[ H3  0  4]"  PolePairs=20  InitialConditions=[0 -46.4509 0.648737 0.648737 0.648737 6.89632 -113.104 126.896 1.29912]  SetSaturation=off  Saturation=[0.6404,0.7127,0.8441,0.9214,0.9956,1.082,1.19,1.316,1.457;0.7,0.7698,0.8872,0.9466,0.9969,1.046,1.1,1.151,1.201]  LoadFlowParameters=[1,0,0,0,0]  TsPowergui=0  TsBlock=-1  IterativeModel=Trapezoidal non iterative  IterativeDiscreteModel=Trapezoidal non iterative  BusType=PV  Pref=85e6  Qref=0  Qmin=-inf  Qmax=inf  PLF=0  QLF=0
      settings: SourceProductName=Simscape Electrical
  Vref3 : Constant  Value=1.025
  A : PMIOPort  Side=Left
  B : PMIOPort  Port=2  Side=Left
  C : PMIOPort  Port=3  Side=Left
  wires:
  Vref3/1 -> M1: Turbine & Regulators/3(Vref1)
  Synchronous Machine pu Standard/1 -> M1: Turbine & Regulators/1(m)
  M1: Turbine & Regulators/2(Vf1) -> Synchronous Machine pu Standard/2
  M1: Turbine & Regulators/1(Pm1) -> Synchronous Machine pu Standard/1
  [PSSmodel] -> M1: Turbine & Regulators/4(PSS1)
  Pref3/1 -> M1: Turbine & Regulators/2(Pref1)
  connections:
  Synchronous Machine pu Standard/RConn3 -- C/RConn1
  Synchronous Machine pu Standard/RConn2 -- B/RConn1
  Synchronous Machine pu Standard/RConn1 -- A/RConn1

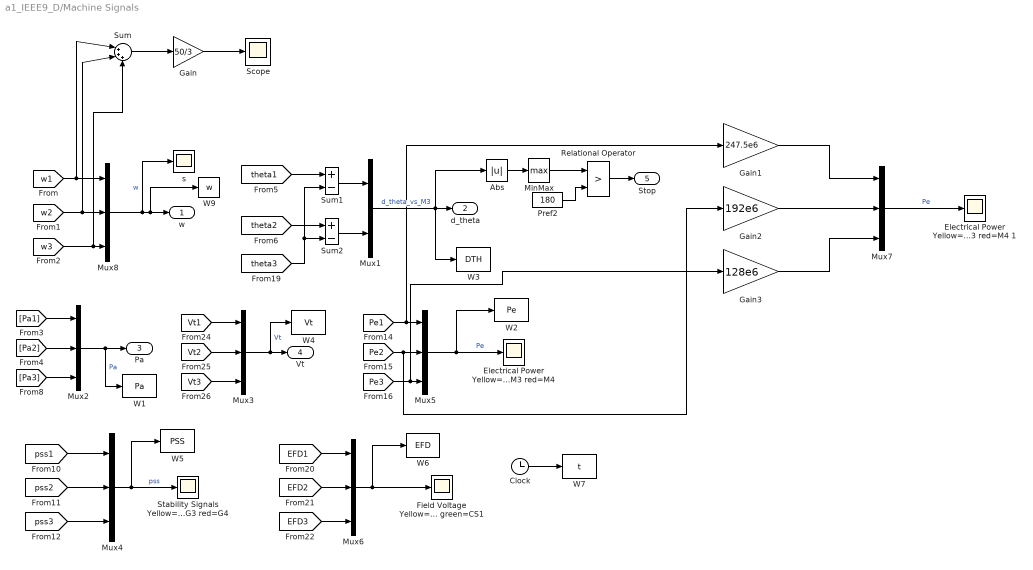
== system a1_IEEE9_D/Machine Signals ==
  Abs : Abs  SaturateOnIntegerOverflow=on
  Clock : Clock
  "Electrical Power Yellow=M1 mag=M2 cyan=M3 red=M4 " : Scope
  Electrical Power Yellow=M1 mag=M2 cyan=M3 red=M4 1 : Scope
  Field Voltage Yellow=G1 mag=G2 cyan=G3 red=G4 green=CS1 : Scope
  Gain : Gain  Gain=50/3
  Gain1 : Gain  Gain=247.5e6
  Gain2 : Gain  Gain=192e6
  Gain3 : Gain  Gain=128e6
  MinMax : MinMax  Function=max  SaturateOnIntegerOverflow=on  InputSameDT=on
  Mux1 : Mux  Inputs=2
  Mux{2..8} (7 alike) : Mux  Inputs=3
  Pref2 : Constant  Value=180
  Relational Operator : RelationalOperator  Operator=>  RndMeth=Nearest  InputSameDT=on
  Scope : Scope
  "Stability Signals Yellow=G1 mag=G2 cyan=G3 red=G4 " : Scope
  Sum : Sum  Inputs=|+++
  Sum1 : Sum  Inputs=+-  SaturateOnIntegerOverflow=on  InputSameDT=on  OutDataTypeStr=Inherit: Same as first input
  Sum2 : Sum  Inputs=+-  SaturateOnIntegerOverflow=on  InputSameDT=on  OutDataTypeStr=Inherit: Same as first input
  W1 : ToWorkspace  VariableName=Pa  SampleTime=1/60
  W2 : ToWorkspace  VariableName=Pe  SampleTime=1/60
  W3 : ToWorkspace  VariableName=DTH  SampleTime=1/60
  W4 : ToWorkspace  VariableName=Vt  SampleTime=1/60
  W5 : ToWorkspace  VariableName=PSS  SampleTime=1/60
  W6 : ToWorkspace  VariableName=EFD  SampleTime=1/60
  W7 : ToWorkspace  VariableName=t  SampleTime=1/60
  W9 : ToWorkspace  VariableName=w  SaveFormat=Timeseries  SampleTime=1/60
  s : Scope
  w : Outport
  d_theta : Outport  Port=2
  Pa : Outport  Port=3
  Vt : Outport  Port=4
  Stop : Outport  Port=5
  wires:
  Mux8/1 -> s/1, W9/1, w/1  "w"
  [w1] -> Sum/1, Mux8/1
  [w2] -> Sum/2, Mux8/2
  [w3] -> Sum/3, Mux8/3
  Mux1/1 -> d_theta/1, Abs/1, W3/1  "d_theta_vs_M3"
  Abs/1 -> MinMax/1
  Pref2/1 -> Relational Operator/2
  MinMax/1 -> Relational Operator/1
  [Pa1] -> Mux2/1
  Mux4/1 -> "Stability Signals Yellow=G1 mag=G2 cyan=G3 red=G4 "/1, W5/1  "pss"
  [pss1] -> Mux4/1
  [pss2] -> Mux4/2
  [pss3] -> Mux4/3
  [EFD1] -> Mux6/1
  [EFD2] -> Mux6/2
  [EFD3] -> Mux6/3
  Mux6/1 -> Field Voltage Yellow=G1 mag=G2 cyan=G3 red=G4 green=CS1/1, W6/1
  Relational Operator/1 -> Stop/1
  Mux2/1 -> Pa/1, W1/1  "Pa"
  [theta1] -> Sum1/1
  Sum1/1 -> Mux1/1
  [theta2] -> Sum2/1
  [theta3] -> Sum1/2, Sum2/2
  Sum2/1 -> Mux1/2
  [Pa2] -> Mux2/2
  [Pa3] -> Mux2/3
  [Vt1] -> Mux3/1
  [Vt2] -> Mux3/2
  [Vt3] -> Mux3/3
  Mux3/1 -> Vt/1, W4/1  "Vt"
  [Pe1] -> Gain1/1, Mux5/1
  [Pe2] -> Gain2/1, Mux5/2
  [Pe3] -> Gain3/1, Mux5/3
  Mux5/1 -> "Electrical Power Yellow=M1 mag=M2 cyan=M3 red=M4 "/1, W2/1  "Pe"
  Clock/1 -> W7/1
  Sum/1 -> Gain/1
  Gain/1 -> Scope/1
  Gain2/1 -> Mux7/2
  Gain1/1 -> Mux7/1
  Gain3/1 -> Mux7/3
  Mux7/1 -> Electrical Power Yellow=M1 mag=M2 cyan=M3 red=M4 1/1  "Pe"

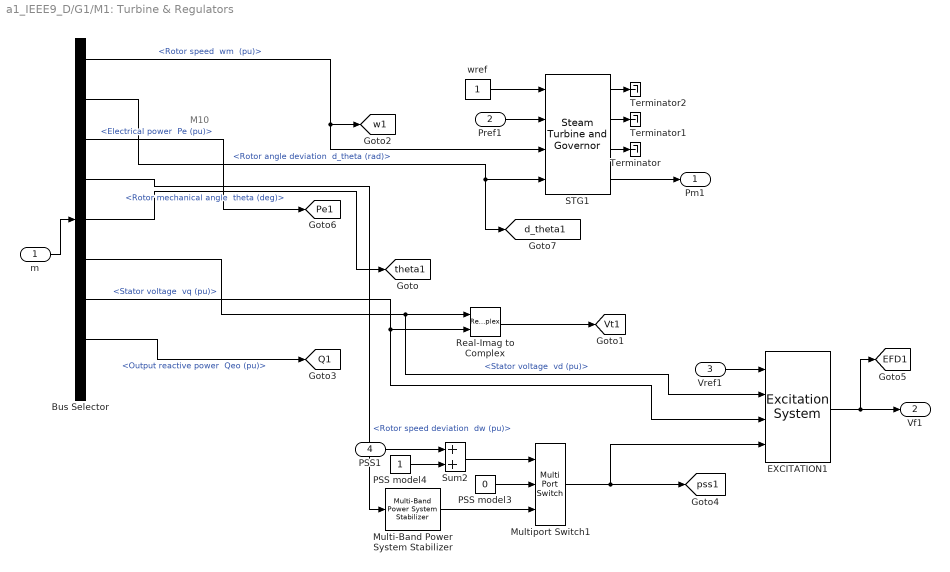
== system a1_IEEE9_D/G1/M1: Turbine & Regulators ==
  note: M10
  m : Inport
  Pref1 : Inport  Port=2
  Vref1 : Inport  Port=3
  PSS1 : Inport  Port=4
  Bus Selector : BusSelector  OutputSignals="Mechanical.Rotor speed  wm  (pu),Mechanical.Rotor angle deviation  d_theta (rad),Mechanical.Electrical power  Pe (pu),Mechanical.Rotor speed deviation  dw (pu),Mechanical.Rotor mechanical angle  theta (deg),dq0 components.Stator voltage  vd (pu),dq0 components.Stator voltage  vq (pu),Output reactive power  Qeo (pu),Output active power   Peo (pu)"
  EXCITATION1 : sps_avr/Excitation System  tr=0.01  reg=[20 0.2 ]  exc=[ 1, 0.314 ]  tgr=[10 1]  damp=[ 0, 0 ]  sat=[ 0, 0 ]  lim="[-5 5  0 ]"  v0=[1.04 1.3869]
      settings: SourceProductName=Simscape Electrical  SourceProductBaseCode=PS
  Multi-Band Power System Stabilizer : powerlib/Machines/Multi-Band Power System Stabilizer  OperationMode=Simplified settings  Kg=k8  GL=[k9 k10]  GI=[k11 k12]  GH=[k13 k14]  GLd=[66 66 9.4]  TcLF=[1.667 2 0 0 0 0 2 2.4 0 0 0 0 1 1]  GId=[66 66 47.6]  TcIF=[1 1 0.25 0.3 0 0 1 1 0.3 0.36 0 0 0 0]  GHd=[66 66 233]  TcHF="[0.01 0.012 0 0 0 0  0.012 0.0144 0 0 0 0 1 1]"  LIM=[.075 .15 .15 .15]  Plot_On=off  MagdB_On=off  FreqRange=logspace(-2,2,500)
      settings: SourceProductName=Simscape Electrical  SourceProductBaseCode=PS
  Multiport Switch1 : MultiPortSwitch  Inputs=2  InputSameDT=on
  PSS model3 : Constant  Value=0
  PSS model4 : Constant
  Real-Imag to Complex : RealImagToComplex
  STG1 : powerlib/Machines/Steam Turbine and Governor  gentype=Tandem-compound (single mass)  reg1="[ 1  R1    0 ]"  reg2="[ 0.001  0.15 ]"  reg3="[ -0.1  0.1  0  4.496 ]"  N=3600  turb1="[ 0  10   3.3   0.5   ]"  turb2="[   0   0.36    0.36   0.28   ]"  HA="[ 0.046  1.430  1.465   0.192 ]"  KA="[ 90.44  53.88  64.59   62.94  ]"  DA="[ 0.0115  0.3575  0.3663   0.0137  ]"  ini1=0.29221  ini2=[0.779316,-31.4247]
      settings: SourceProductName=Simscape Electrical  SourceProductBaseCode=PS
  Sum2 : Sum  SaturateOnIntegerOverflow=on  InputSameDT=on  OutDataTypeStr=Inherit: Same as first input
  Terminator : Terminator
  Terminator1 : Terminator
  Terminator2 : Terminator
  wref : Constant
  Pm1 : Outport  InitialOutput=0
  Vf1 : Outport  Port=2  InitialOutput=0
  tag scope: EFD1=global, Pe1=global, Q1=global, Vt1=global, d_theta1=global, pss1=global, theta1=global, w1=global
  wires:
  Bus Selector/7 -> EXCITATION1/3, Real-Imag to Complex/2  "<Stator voltage  vq (pu)>"
  wref/1 -> STG1/1
  Pref1/1 -> STG1/2
  m/1 -> Bus Selector/1
  Vref1/1 -> EXCITATION1/1
  EXCITATION1/1 -> Vf1/1, [EFD1]
  Real-Imag to Complex/1 -> [Vt1]
  Bus Selector/5 -> [theta1]  "<Rotor mechanical angle  theta (deg)>"
  Bus Selector/6 -> EXCITATION1/2, Real-Imag to Complex/1  "<Stator voltage  vd (pu)>"
  STG1/3 -> Terminator/1
  STG1/4 -> Pm1/1
  STG1/2 -> Terminator1/1
  STG1/1 -> Terminator2/1
  Bus Selector/1 -> STG1/3, [w1]  "<Rotor speed  wm  (pu)>"
  Bus Selector/2 -> [d_theta1], STG1/4  "<Rotor angle deviation  d_theta (rad)>"
  Bus Selector/3 -> [Pe1]  "<Electrical power  Pe (pu)>"
  Bus Selector/8 -> [Q1]  "<Output reactive power  Qeo (pu)>"
  PSS1/1 -> Sum2/1
  Sum2/1 -> Multiport Switch1/1
  PSS model4/1 -> Sum2/2
  Multi-Band Power System Stabilizer/1 -> Multiport Switch1/3
  PSS model3/1 -> Multiport Switch1/2
  Multiport Switch1/1 -> [pss1], EXCITATION1/4
  Bus Selector/4 -> Multi-Band Power System Stabilizer/1  "<Rotor speed deviation  dw (pu)>"

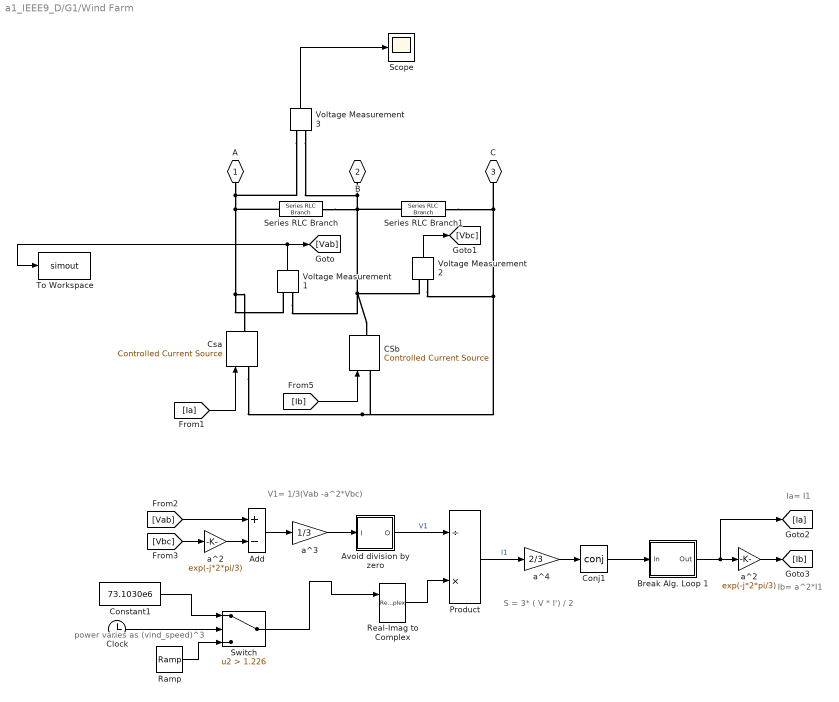
== system a1_IEEE9_D/G1/Wind Farm ==
  note: power varies as (vind_speed)^3
  note: V1= 1/3(Vab -a^2*Vbc)
  note: S = 3* ( V * I') / 2
  note: Ia= I1
  note: Ib= a^2*I1
  Add : Sum  Inputs=+-
  Avoid division by zero : Subsystem
  Break Alg. Loop 1 : Subsystem
  CSb : powerlib/Electrical Sources/Controlled Current Source  Initialize=on  Source_Type=AC  Amplitude=0  Phase=(-0.5-2*pi/3)*180/pi  Frequency=60  Measurements=Current
      settings: SourceProductName=Simscape Electrical
  Clock : Clock
  Conj1 : Math  Operator=conj  SaturateOnIntegerOverflow=on
  Constant1 : Constant  Value=73.1030e6
  Csa : powerlib/Electrical Sources/Controlled Current Source  Initialize=on  Source_Type=AC  Amplitude=0  Phase=-0.5*180/pi  Frequency=50  Measurements=Current
      settings: SourceProductName=Simscape Electrical
  Product : Product  Inputs=/*  SaturateOnIntegerOverflow=on  InputSameDT=on  OutDataTypeStr=Inherit: Same as first input
  Ramp : simulink/Sources/Ramp  slope=59.62727e6  start=0  InitialOutput=0
  Real-Imag to Complex : RealImagToComplex
  Scope : Scope
  Series RLC Branch : powerlib/Elements/Series RLC Branch  LConnTagsString=__new0  RConnTagsString=__new0  BranchType=R  Resistance=1e6  Inductance=1e-3  SetiL0=off  InitialCurrent=0  Capacitance=1e-6  Setx0=off  InitialVoltage=0  Measurements=None
      settings: SourceProductName=Simscape Electrical
  Series RLC Branch1 : powerlib/Elements/Series RLC Branch  LConnTagsString=__new0  RConnTagsString=__new0  BranchType=R  Resistance=1e6  Inductance=1e-3  SetiL0=off  InitialCurrent=0  Capacitance=1e-6  Setx0=off  InitialVoltage=0  Measurements=None
      settings: SourceProductName=Simscape Electrical
  Switch : Switch  Criteria=u2 > Threshold  Threshold=1.226
  To Workspace : ToWorkspace  VariableName=simout  SaveFormat=Timeseries  SampleTime=-1
  Voltage Measurement1 : powerlib/Measurements/Voltage Measurement  PhasorSimulation=on  OutputType=Complex  PSBequivalent=0
      settings: SourceProductName=Simscape Electrical
  Voltage Measurement2 : powerlib/Measurements/Voltage Measurement  PhasorSimulation=on  OutputType=Complex  PSBequivalent=0
      settings: SourceProductName=Simscape Electrical
  Voltage Measurement3 : powerlib/Measurements/Voltage Measurement  PhasorSimulation=on  OutputType=Magnitude  PSBequivalent=0
      settings: SourceProductName=Simscape Electrical
  a^2 : Gain  Gain=exp(-j*2*pi/3)  SaturateOnIntegerOverflow=on  OutDataTypeStr=Inherit: Same as input  ParamDataTypeStr=Inherit: Same as input
  "a^2 " : Gain  Gain=exp(-j*2*pi/3)  SaturateOnIntegerOverflow=on  OutDataTypeStr=Inherit: Same as input  ParamDataTypeStr=Inherit: Same as input
  a^3 : Gain  Gain=1/3  SaturateOnIntegerOverflow=on  OutDataTypeStr=Inherit: Same as input  ParamDataTypeStr=Inherit: Same as input
  a^4 : Gain  Gain=2/3  SaturateOnIntegerOverflow=on  OutDataTypeStr=Inherit: Same as input  ParamDataTypeStr=Inherit: Same as input
  A : PMIOPort  Tag=PMCPort  Side=Right
  B : PMIOPort  Tag=PMCPort  Port=2  Side=Right
  C : PMIOPort  Tag=PMCPort  Port=3  Side=Right
  wires:
  "a^2 "/1 -> Add/2
  [Vbc] -> "a^2 "/1
  Avoid division by zero/1(O) -> Product/1  "V1"
  a^3/1 -> Avoid division by zero/1(I)
  Add/1 -> a^3/1
  [Vab] -> Add/1
  Voltage Measurement1/1 -> To Workspace/1, [Vab]
  Voltage Measurement2/1 -> [Vbc]
  Real-Imag to Complex/1 -> Product/2
  Product/1 -> a^4/1  "I1"
  a^2/1 -> [Ib]
  a^4/1 -> Conj1/1
  Conj1/1 -> Break Alg. Loop 1/1(In)
  Break Alg. Loop 1/1(Out) -> [Ia], a^2/1
  Switch/1 -> Real-Imag to Complex/1
  [Ib] -> CSb/1
  [Ia] -> Csa/1
  Ramp/1 -> Switch/3
  Constant1/1 -> Switch/1
  Clock/1 -> Switch/2
  Voltage Measurement3/1 -> Scope/1
  connections:
  A/RConn1 -- Voltage Measurement3/LConn1 -- Csa/RConn1 -- Voltage Measurement1/LConn1 -- Series RLC Branch/LConn1
  Voltage Measurement2/LConn2 -- Series RLC Branch1/RConn1 -- C/RConn1 -- CSb/LConn1 -- Csa/LConn1
  CSb/RConn1 -- Series RLC Branch/RConn1 -- Voltage Measurement3/LConn2 -- B/RConn1 -- Series RLC Branch1/LConn1 -- Voltage Measurement2/LConn1 -- Voltage Measurement1/LConn2

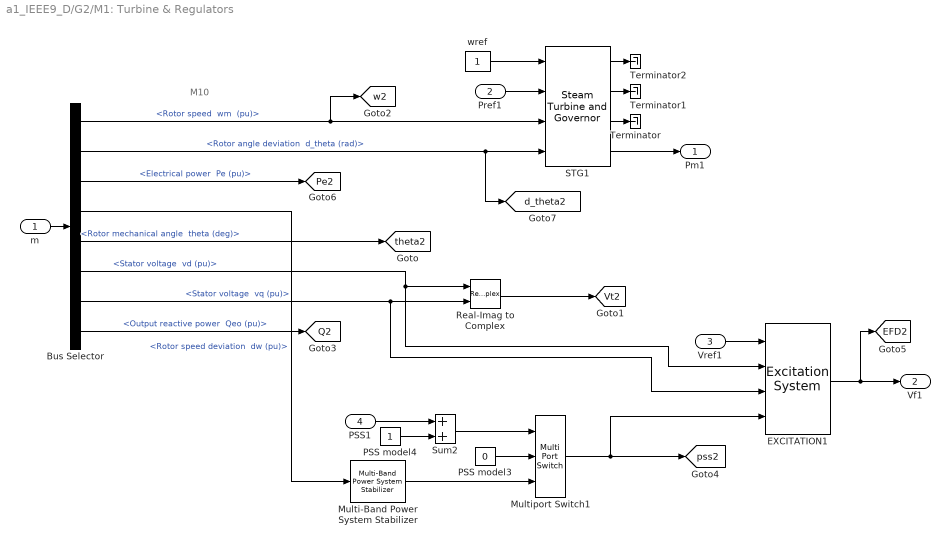
== system a1_IEEE9_D/G2/M1: Turbine & Regulators ==
  note: M10
  m : Inport
  Pref1 : Inport  Port=2
  Vref1 : Inport  Port=3
  PSS1 : Inport  Port=4
  Bus Selector : BusSelector  OutputSignals="Mechanical.Rotor speed  wm  (pu),Mechanical.Rotor angle deviation  d_theta (rad),Mechanical.Electrical power  Pe (pu),Mechanical.Rotor speed deviation  dw (pu),Mechanical.Rotor mechanical angle  theta (deg),dq0 components.Stator voltage  vd (pu),dq0 components.Stator voltage  vq (pu),Output reactive power  Qeo (pu)"
  EXCITATION1 : sps_avr/Excitation System  tr=0.01  reg=[ 20 .2 ]  exc=[ 1, 0.314 ]  tgr="[10    1]"  damp=[ 0.63, 0.35 ]  sat=[ 0, 0 ]  lim=[ -5 5 0 ]  v0=[1.025 1.2464]
      settings: SourceProductName=Simscape Electrical  SourceProductBaseCode=PS
  Multi-Band Power System Stabilizer : powerlib/Machines/Multi-Band Power System Stabilizer  OperationMode=Simplified settings  Kg=k15  GL=[k16 k17]  GI=[k18 k19]  GH=[k20 k21]  GLd=[66 66 9.4]  TcLF=[1.667 2 0 0 0 0 2 2.4 0 0 0 0 1 1]  GId=[66 66 47.6]  TcIF=[1 1 0.25 0.3 0 0 1 1 0.3 0.36 0 0 0 0]  GHd=[66 66 233]  TcHF="[0.01 0.012 0 0 0 0  0.012 0.0144 0 0 0 0 1 1]"  LIM=[.075 .15 .15 .15]  Plot_On=off  MagdB_On=off  FreqRange=logspace(-2,2,500)
      settings: SourceProductName=Simscape Electrical  SourceProductBaseCode=PS
  Multiport Switch1 : MultiPortSwitch  Inputs=2  InputSameDT=on
  PSS model3 : Constant  Value=0
  PSS model4 : Constant
  Real-Imag to Complex : RealImagToComplex
  STG1 : powerlib/Machines/Steam Turbine and Governor  gentype=Tandem-compound (single mass)  reg1="[ 1  R2    0 ]"  reg2="[ 0.001  0.15 ]"  reg3="[ -0.1  0.1  0  4.496 ]"  N=3600  turb1="[ 0  10   3.3   0.5   ]"  turb2="[   0   0.36    0.36   0.28   ]"  HA="[ 0.046  1.430  1.465   0.192 ]"  KA="[ 90.44  53.88  64.59   62.94  ]"  DA="[ 0.0115  0.3575  0.3663   0.0137  ]"  ini1=0.85068  ini2=[0.779316,-31.4247]
      settings: SourceProductName=Simscape Electrical  SourceProductBaseCode=PS
  Sum2 : Sum  SaturateOnIntegerOverflow=on  InputSameDT=on  OutDataTypeStr=Inherit: Same as first input
  Terminator : Terminator
  Terminator1 : Terminator
  Terminator2 : Terminator
  wref : Constant
  Pm1 : Outport  InitialOutput=0
  Vf1 : Outport  Port=2  InitialOutput=0
  tag scope: EFD2=global, Pe2=global, Q2=global, Vt2=global, d_theta2=global, pss2=global, theta2=global, w2=global
  wires:
  Bus Selector/7 -> EXCITATION1/3, Real-Imag to Complex/2  "<Stator voltage  vq (pu)>"
  wref/1 -> STG1/1
  Pref1/1 -> STG1/2
  m/1 -> Bus Selector/1
  Vref1/1 -> EXCITATION1/1
  EXCITATION1/1 -> Vf1/1, [EFD2]
  Real-Imag to Complex/1 -> [Vt2]
  Bus Selector/5 -> [theta2]  "<Rotor mechanical angle  theta (deg)>"
  Bus Selector/6 -> Real-Imag to Complex/1, EXCITATION1/2  "<Stator voltage  vd (pu)>"
  STG1/3 -> Terminator/1
  STG1/4 -> Pm1/1
  STG1/2 -> Terminator1/1
  STG1/1 -> Terminator2/1
  Bus Selector/1 -> [w2], STG1/3  "<Rotor speed  wm  (pu)>"
  Bus Selector/2 -> [d_theta2], STG1/4  "<Rotor angle deviation  d_theta (rad)>"
  Bus Selector/3 -> [Pe2]  "<Electrical power  Pe (pu)>"
  Bus Selector/8 -> [Q2]  "<Output reactive power  Qeo (pu)>"
  PSS1/1 -> Sum2/1
  Sum2/1 -> Multiport Switch1/1
  PSS model4/1 -> Sum2/2
  Multi-Band Power System Stabilizer/1 -> Multiport Switch1/3
  PSS model3/1 -> Multiport Switch1/2
  Multiport Switch1/1 -> [pss2], EXCITATION1/4
  Bus Selector/4 -> Multi-Band Power System Stabilizer/1  "<Rotor speed deviation  dw (pu)>"
